simulink model "Custom_SP_inverse"  (R2020b)
settings: Solver=ode45  StartTime=0.0  StopTime=40  RelTol=1e-3
model workspace (MATLAB code in the model file):
  | %% PARAMETERS FOR CUSTOM_SP
  | %%%%%%%%%%%%%%%%%%%%% DENSITY %%%%%%%%%%%%%%%%%%%%%%%
  | al = 2.07; % g/cm^3
  | steel = 7.833; %g/cm^3
  | 
  | %%%%%%%%%%%%%%%%%%%%% BASE COORDINATES %%%%%%%%%%%%%%%%%%%%%%%
  | % Outside coordinates
  | out_base_right = [-335 -170.32; -315 -204.96;
  |     -315 -295.6; -98.49 -420.6; -20 -375.28;
  |     20 -375.28; 315 -204.96; 335 -170.32; 413.49 -125];
  | out_base_left = [413.49 125; 335 170.32;
  |     315 204.96; 20 375.28; -20 375.28;
  |     -98.49 420.6; -315 295.6; -315 204.96; -335 170.32;
  |     -335 -170.32];
  | out_base = [out_base_right; out_base_left];
  | 
  | % Inside coordinates
  | in_base = [-230 -246.52; -230 246.52; -98.49 322.45; 328.49 75.93;
  |     328.49 -75.93; -98.49 -322.45; -230 -246.52];
  | 
  | tot_base = [out_base; in_base];
  | 
  | %%%%%%%%%%%%%%%%%%%%%%% PLATE POSE ON BASE %%%%%%%%%%%%%%%%%%%%%%%%%%%
  | % PLATE POSITION ON BASE
  | plate_1 = [-272.22 -252.09 0];
  | plate_2 = [-82.21 -361.79 0];
  | plate_3 = [354.42 -109.71 0];
  | plate_4 = [354.42 109.71 0];
  | plate_5 = [-82.21 361.79 0];
  | plate_6 = [-272.22  252.09 0];
  | 
  | % ANGLE FOR JOINT ON BASE
  | plate_angle_1 = 0 + pi/2;
  | plate_angle_2 = 2*pi/3 + pi/2;
  | plate_angle_3 = 2*pi/3 + pi/2;
  | plate_angle_4 = 4*pi/3 + pi/2;
  | plate_angle_5 = 4*pi/3 + pi/2;
  | plate_angle_6 = 0 + pi/2;
  | 
  | %%%%%%%%%%%%%%%%%%%%%%%% FLANGE COORDINATES %%%%%%%%%%%%%%%%%%%%%%%%%%%%
  | flange_body = [ -20 22.5; -20 -22.5; 13.6488 -9.3106];
  | 
  | C = linspace(-68.6, 68.6, 21)';
  | C = deg2rad(C);
  | flange_round = [10+10*cos(C) 10*sin(C)];
  | 
  | C = linspace(3*pi/2, -pi/2, 100)';
  | flange_hole = [10+6*cos(C) 6*sin(C)];
  | 
  | flange = [flange_round; flange_body; flange_hole];
  | 
  | %plot(flange(:,1),flange(:,2), 'Color', [0.6 0.6 0.6], 'Marker', '.',...
  | %'MarkerSize', 9, 'MarkerEdgeColor', [1 0 0]);
  | 
  | %%%%%%%%%%%%%%%%%%%%%%%%%%%%% LID %%%%%%%%%%%%%%%%%%%%%%%%%%%%%%
  | % LID COORDINATES
  | C = linspace(-150 , -70, 9)';
  | C = deg2rad(C);
  | lid_round1 = [-171.37+10*cos(C) -103.18+10*sin(C)];
  | 
  | C = linspace(110, 60, 9)';
  | C = deg2rad(C);
  | lid_round2 = [-118.05+10*cos(C) -105.05+10*sin(C)];
  | 
  | C = linspace(60, 10, 9)';
  | C = deg2rad(C);
  | lid_round3 = [-117.46+10*cos(C) -105.39+10*sin(C)];
  | 
  | C = linspace(110, 60, 9)';
  | C = deg2rad(C);
  | lid_round4 = [-32.54+10*cos(C) -154.42+10*sin(C)];
  | 
  | C = linspace(60, 10, 9)';
  | C = deg2rad(C);
  | lid_round5 = [-31.95+10*cos(C) -154.76+10*sin(C)];
  | 
  | C = linspace(-90-80, -90, 9)';
  | C = deg2rad(C);
  | lid_round6 = [-3.67+10*cos(C) -200+10*sin(C)];
  | 
  | C = linspace(-30, 50, 9)';
  | C = deg2rad(C);
  | lid_round7 = [175.04+10*cos(C) -96.82+10*sin(C)];
  | 
  | C = linspace(-140, -90, 9)';
  | C = deg2rad(C);
  | lid_round8 = [150+10*sin(C) -49.71+10*cos(C)];
  | 
  | C = linspace(-90, -40, 9)';
  | C = deg2rad(C);
  | lid_round9 = [150+10*sin(C) -49.03+10*cos(C)];
  | 
  | C = linspace(-140, -90, 9)';
  | C = deg2rad(C);
  | lid_round10 = [150+10*sin(C) 49.03+10*cos(C)];
  | 
  | C = linspace(-90, -40, 9)';
  | C = deg2rad(C);
  | lid_round11 = [150+10*sin(C) 49.71+10*cos(C)];
  | 
  | C = linspace(-50, 30, 9)';
  | C = deg2rad(C);
  | lid_round12 = [175.04+10*cos(C) 96.82+10*sin(C)];
  | 
  | C = linspace(90, 90+80, 9)';
  | C = deg2rad(C);
  | lid_round13 = [-3.67+10*cos(C) 200+10*sin(C)];
  | 
  | C = linspace(-10, -60, 9)';
  | C = deg2rad(C);
  | lid_round14 = [-31.95+10*cos(C) 154.76+10*sin(C)];
  | 
  | C = linspace(-60, -110, 9)';
  | C = deg2rad(C);
  | lid_round15 = [-32.54+10*cos(C) 154.42+10*sin(C)];
  | 
  | C = linspace(-10, -60, 9)';
  | C = deg2rad(C);
  | lid_round16 = [-117.46+10*cos(C) 105.39+10*sin(C)];
  | 
  | C = linspace(-60, -110, 9)';
  | C = deg2rad(C);
  | lid_round17 = [-118.05+10*cos(C) 105.05+10*sin(C)];
  | 
  | C = linspace(70 , 150, 9)';
  | C = deg2rad(C);
  | lid_round18 = [-171.37+10*cos(C) 103.18+10*sin(C)];
  | 
  | lid = [-200 -73.59; lid_round1; lid_round2;
  |     lid_round3;
  |     -100.49 -144.05; -74.51 -159.05; lid_round4;
  |     lid_round5; lid_round6; 36.27 -210; 163.73 -136.41;
  |     lid_round7; lid_round8; lid_round9; 175 -15; 175 15;
  |     lid_round10; lid_round11; lid_round12; 163.73 136.41;
  |     36.27 210; lid_round13; lid_round14; lid_round15;
  |     -74.51 159.05; -100.49 144.05; lid_round16;
  |     lid_round17; lid_round18; -200 73.59];
  | 
  | lid = [-200 -73.59; lid_round1; lid_round2; lid_round3;
  |     -100.49 -144.05; -74.51 -159.05;
  |     lid_round4; lid_round5; lid_round6;
  |     36.27 -210; 163.73 -136.41;
  |     lid_round7; lid_round8; lid_round9;
  |     175 -15; 175 15;
  |     lid_round10; lid_round11; lid_round12;
  |     163.73 136.41; 36.27 210;
  |     lid_round13; lid_round14; lid_round15;
  |     -74.51 159.05; -100.49 144.05;
  |     lid_round16; lid_round17; lid_round18; -200 73.59];
  | 
  | % LID CONNECTOR
  | C = linspace(-150 , -50, 15)';
  | C = deg2rad(C);
  | lid_connector_round1 = [2.15+10*cos(C) -79.37+10*sin(C)];
  | 
  | C = linspace(-50 , 0, 15)';
  | C = deg2rad(C);
  | lid_connector_round2 = [37.5+10*cos(C) -49.71+10*sin(C)];
  | 
  | C = linspace(0 , 50, 15)';
  | C = deg2rad(C);
  | lid_connector_round3 = [37.5+10*cos(C) -49.03+10*sin(C)];
  | 
  | C = linspace(-50, 0, 15)';
  | C = deg2rad(C);
  | lid_connector_round4 = [37.5+10*cos(C) 49.03+10*sin(C)];
  | 
  | C = linspace(0, 50, 15)';
  | C = deg2rad(C);
  | lid_connector_round5 = [37.5+10*cos(C) 49.71+10*sin(C)];
  | 
  | C = linspace(50 , 150, 15)';
  | C = deg2rad(C);
  | lid_connector_round6 = [2.15+10*cos(C) 79.37+10*sin(C)];
  | 
  | lid_connector = [-12.5 -74; lid_connector_round1;
  |     lid_connector_round2; lid_connector_round3; 12.5 -15;
  |     12.5 15; lid_connector_round4; lid_connector_round5;
  |     lid_connector_round6; -12.5 74];
  | 
  | %%%%%%%%%%%%%%%%%%%%%%%%% BALL JOINT %%%%%%%%%%%%%%%%%%%%%%%%%%%
  | % BALL JOINTS
  | C = linspace(138.59, 41.41, 50)';
  | C = deg2rad(C);
  | ball_round = [10*sin(C) 10*cos(C)];
  | 
  | ball_joint = [6 -7.5; ball_round; 6 7.5];
  | 
  | % BALL CONNECTOR
  | C = linspace(-109.47, -70.53, 49)';
  | C = deg2rad(C);
  | ball_round_out = [-16*sin(C) 16*cos(C)];
  | 
  | C = linspace(-57.75, -122.25, 49)';
  | C = deg2rad(C);
  | ball_round_in = [-10*sin(C) 10*cos(C)];
  | 
  | ball_connector = [ball_round_out; ball_round_in];
  | 
  | %%%%%%%%%%%%%%%%%%%%%%%%%% MOTOR %%%%%%%%%%%%%%%%%%%%%%%%%%%
  | % KNOB UNDER MOTOR
  | C = linspace(-90+25.84, -90+64.16, 50)';
  | C = deg2rad(C);
  | knob_under_round1 = [7.5*sin(C) -7.5*cos(C)];
  | 
  | C = linspace( -64.16, -25.84, 50)';
  | C = deg2rad(C);
  | knob_under_round2 = [7.5*cos(C) 7.5*sin(C)];
  | 
  | C = linspace( 25.84, 64.16, 50)';
  | C = deg2rad(C);
  | knob_under_round3 = [7.5*cos(C) 7.5*sin(C)];
  | 
  | C = linspace( 64.16, 25.84, 50)';
  | C = deg2rad(C);
  | knob_under_round4 = [-7.5*cos(C) 7.5*sin(C)];
  | 
  | knob_under = [knob_under_round1; knob_under_round2;
  |     knob_under_round3; knob_under_round4];
  | 
  | % MOTOR UNDER
  | C = linspace(-90, -49, 10)';
  | C = deg2rad(C);
  | knob_under_round1 = [-(19+17)+5.5*sin(C) -11.13-5.5*cos(C)];
  | 
  | C = linspace(-49, 0, 10)';
  | C = deg2rad(C);
  | knob_under_round2 = [-(17+14.77)+5.5*sin(C) -16-5.5*cos(C)];
  | 
  | C = linspace(0, 180, 49)';
  | C = deg2rad(C);
  | knob_under_round3 = [20+21.5*sin(C) -21.5*cos(C)];
  | 
  | C = linspace(180, 180+49, 10)';
  | C = deg2rad(C);
  | knob_under_round4 = [-(17+14.77)+5.5*sin(C) 16-5.5*cos(C)];
  | 
  | C = linspace(270-49, 270, 10)';
  | C = deg2rad(C);
  | knob_under_round5 = [-(19+17)+5.5*sin(C) 11.13-5.5*cos(C)];
  | 
  | motor_under = [knob_under_round1; knob_under_round2;
  |     knob_under_round3; knob_under_round4; knob_under_round5];
  | 
  | % MOTOR LINEAR
  | C = linspace(-180, -101.99, 10)';
  | C = deg2rad(C);
  | motor_top_round1 = [-15.28+3*cos(C) -8.62+3*sin(C)];
  | 
  | C = linspace(-101.99, 101.99, 49)';
  | C = deg2rad(C);
  | motor_top_round2 = [3.12+15.25*cos(C) 15.25*sin(C)];
  | 
  | C = linspace(101.99, 180, 10)';
  | C = deg2rad(C);
  | motor_top_round3 = [-15.28+3*cos(C) 8.62+3*sin(C)];
  | 
  | C = linspace(180, -180, 50)';
  | C = deg2rad(C);
  | motor_top_hole = [3.12+10.1*cos(C) 10.1*sin(C)];
  | 
  | motor_linear = [motor_top_round1; motor_top_round2; motor_top_round3;
  |     -15.28-3 -8.62; motor_top_hole];
  | 
  | %%%%%%%%%%%%%%%%%%%%% MALE %%%%%%%%%%%%%%%%%%%%%%%%%%%
  | male = [15.1 -16; 15.1 16; 10.1 16;
  |     10.1 -11; 6 -11; 6 -16];
  | 
  | %%%%%%%%%%%%%%%%%%%%% FEMALE %%%%%%%%%%%%%%%%%%%%%%%%%
  | female = [15 -19; 15 19; 9.5 19; 9.5 1;
  |     5.055 1; 5.055 -19];
  | 
  | %%%%%%%%%%%%%%%%%%%%% STRAIN GAUGE %%%%%%%%%%%%%%%%%%%%%%
  | strain_gauge = [-38.1 -25.4; -22.4 -25.4; -22.4 11.6;
  |     -13.9 11.6; -13.9 -25.4; 38.1 -25.4; 38.1 25.4;
  |     22.4 25.4; 22.4 -11.6; 13.9 -11.6;
  |     13.9 25.4; -38.1 25.4];
  | 
  | %%%%%%%%%%%%%%%%%%%%% M12 STUFF %%%%%%%%%%%%%%%%%%%%%%%%%%%
  | % M12 BOLT
  | m12_bolt = [0 -18.5; 6 -18.5; 6 11.5; 10.1 11.5; 10.1 18.5; 0 18.5];
  | 
  | % M12 NUT
  | C = linspace(3*pi, pi, 50)';
  | m12_hole = [6*cos(C) 6*sin(C)];
  | m12_nut = [-21.2/2 0; -5.48 -9.5; 5.48 -9.5; 21.2/2 0; 5.48 9.5; -5.48 9.5; -21.2/2 0; m12_hole];
  | 
  | % M12 WASHER
  | m12_washer = [6 -1; 23.5/2 -1; 23.5/2 1; 6 1];
  | 
  | %%%%%%%%%%%%%%%%%%%%%% PLATFORM COORDINATES %%%%%%%%%%%%%%%%%%%%%%%%%%%
  | % Outside coordinates
  | out_platform = [36.27 -210; 163.73 -136.41;
  |     200 -73.59; 200 73.59; 163.73 136.41;
  |     36.27 210; -36.27 210; -163.73 136.41;
  |     -200 73.59; -200 -73.54; -163.73 -136.41; -36.27 -210;
  |     36.27 -210];
  | C = linspace(3*pi/2, -pi/2, 100)';
  | platform_hole = [140*cos(C) 140*sin(C)];
  | platform = [out_platform; platform_hole];
  | 
  | %%%%%%%%%%%%%%%%%%%% STUMP %%%%%%%%%%%%%%%%%%%%%%%
  | C = linspace(-pi/2, -deg2rad(12.47), 100)';
  | stump_round = [70*cos(C) -100+70*sin(C)];
  | stump = [stump_round; 100 170; 0 170];
  | 
  | %% POSITION OF BASE JOINT AND PLATFORM JOINT FOR INVERSE KINEMATICS
  | % BASE JOINT POSITION
  | 
  | zb = 5 + 5 + 30;
  | B = [plate_1(1,1:2) zb; plate_2(1,1:2) zb; plate_3(1,1:2) zb; plate_4(1,1:2) zb; plate_5(1,1:2) zb; plate_6(1,1:2) zb]';
  | 
  | 
  | % JOINT POSITION ON PLATFORM
  | Rot = [cos(deg2rad(120)) -sin(deg2rad(120)); sin(deg2rad(120)) cos(deg2rad(120))];
  | platform_joint_1 = [-200.54-18.5 -48.83]';
  | platform_joint_6 = [-200.54-18.5 48.83]';
  | platform_joint_2 = Rot*platform_joint_6;
  | platform_joint_3 = Rot*platform_joint_1;
  | platform_joint_4 = Rot*platform_joint_2;
  | platform_joint_5 = Rot*platform_joint_3;
  | 
  | % LEG LENGHT AT HOME POSITION
  | %ball_joint_bottom_length = 13.75; %mm
  | %nut_washer = 10 + 2 + 7.25; %mm
  | %female_length = 38 + 2; %mm
  | %motor_length = 58.5 + 163.5; %mm
  | %extender_length = 20 + 50; %mm
  | %male_bolt_nut = 5 + 7 + 25; %mm
  | %strain_gauge_length = 38.1*2; %mm
  | %nut = 10 + 7.25; %mm
  | %ball_joint_top_length = 13.75; %mm
  | 
  | %leg_initial_length = ball_joint_bottom_length + nut_washer + female_length + motor_length + extender_length + male_bolt_nut + strain_gauge_length + nut + ball_joint_top_length;
  | 
  | %height_home = sqrt(leg_initial_length^2 - (plate_1(1)-platform_joint_1(1))^2 - (plate_1(2)-platform_joint_1(2))^2)+zb;
  | height_home = 503.318 + 2.5;
  | leg_initial_length = sqrt((plate_1(1)-platform_joint_1(1))^2 + (plate_1(2)-platform_joint_1(2))^2 + (height_home-zb)^2);
  | P = [platform_joint_1' height_home; platform_joint_2' height_home; platform_joint_3' height_home; platform_joint_4' height_home; platform_joint_5' height_home; platform_joint_6' height_home]';
libraries: nesl_utility x19, Custom_SP_lib x8, sm_lib x2
(part 1 of 2)
settings Model: Creator=ellen  LastModifiedBy=ellen
settings DataIOCC: LimitDataPoints=on

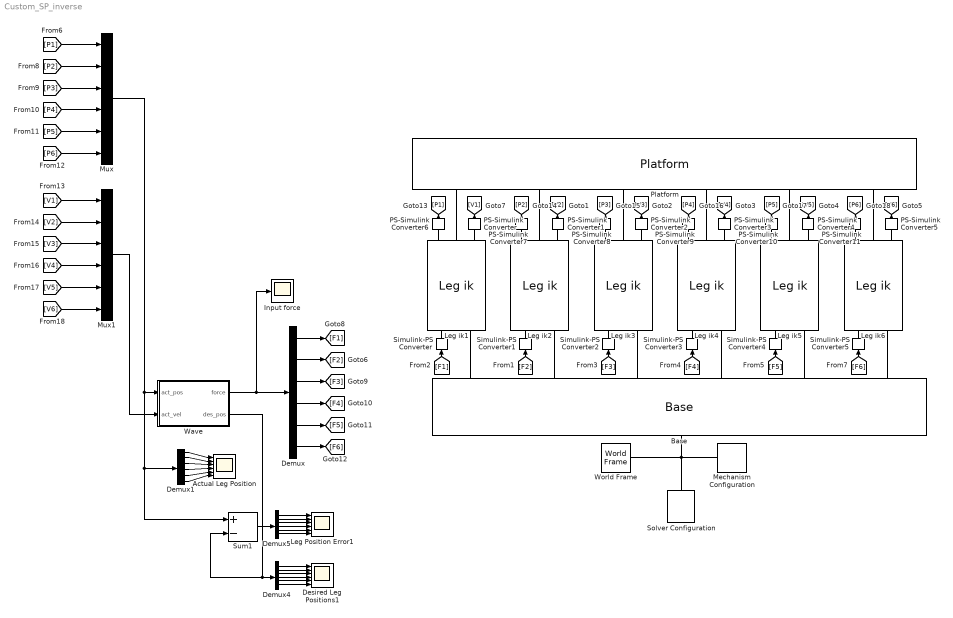
== system Custom_SP_inverse ==
  Actual Leg Position : Scope  NumInputPorts=6
  Base : Custom_SP_lib/Base  SystemSampleTime=-1  VariantActivationTime=update diagram  Latency=0  AutoFrameSizeCalculation=off
  Demux{,1,4..5} (4 alike) : Demux  Outputs=6
  Desired Leg Positions1 : Scope  NumInputPorts=6
  Input force : Scope
  Leg Position Error1 : Scope  NumInputPorts=6
  Leg ik1 : Custom_SP_lib/Leg ik  SystemSampleTime=-1  VariantActivationTime=update diagram  Latency=0  AutoFrameSizeCalculation=off
      link override Motor ik1: leg_offset=0
      link override Motor ik1/Actuation: PositionTargetValue=0
  Leg ik2 : Custom_SP_lib/Leg ik  SystemSampleTime=-1  VariantActivationTime=update diagram  Latency=0  AutoFrameSizeCalculation=off
      link override Motor ik1: leg_offset=0
      link override Motor ik1/Actuation: PositionTargetValue=0
  Leg ik3 : Custom_SP_lib/Leg ik  SystemSampleTime=-1  VariantActivationTime=update diagram  Latency=0  AutoFrameSizeCalculation=off
      link override Motor ik1: leg_offset=0
      link override Motor ik1/Actuation: PositionTargetValue=0
  Leg ik4 : Custom_SP_lib/Leg ik  SystemSampleTime=-1  VariantActivationTime=update diagram  Latency=0  AutoFrameSizeCalculation=off
      link override Motor ik1: leg_offset=0
      link override Motor ik1/Actuation: PositionTargetValue=0
  Leg ik5 : Custom_SP_lib/Leg ik  SystemSampleTime=-1  VariantActivationTime=update diagram  Latency=0  AutoFrameSizeCalculation=off
      link override Motor ik1: leg_offset=0
      link override Motor ik1/Actuation: PositionTargetValue=0
  Leg ik6 : Custom_SP_lib/Leg ik  SystemSampleTime=-1  VariantActivationTime=update diagram  Latency=0  AutoFrameSizeCalculation=off
      link override Motor ik1: leg_offset=0
      link override Motor ik1/Actuation: PositionTargetValue=0
  Mechanism Configuration : sm_lib/Utilities/Mechanism Configuration  UniformGravity=Constant  GravityVector=[0 0 -9.81]  GravityVectorUnits=m/s^2  GravityUnits=m/s^2  LinearizationDelta=0.001  JointModeTransitionNonlinearIterations=2
  Mux : Mux  Inputs=6
  Mux1 : Mux  Inputs=6
  PS-Simulink Converter{,1..5} (6 alike) : nesl_utility/PS-Simulink Converter  PhysicalDomain=network_engine_domain  SubClassName=ps_output  LeftPortType=input  RightPortType=output  PseudoPeriodic=off  Frequencies=[]  Unit=mm/s  AffineConversion=off
  PS-Simulink Converter{6..11} (6 alike) : nesl_utility/PS-Simulink Converter  PhysicalDomain=network_engine_domain  SubClassName=ps_output  LeftPortType=input  RightPortType=output  PseudoPeriodic=off  Frequencies=[]  Unit=mm  AffineConversion=off
  Platform : Custom_SP_lib/Platform  SystemSampleTime=-1  VariantActivationTime=update diagram  Latency=0  AutoFrameSizeCalculation=off
  Simulink-PS Converter{,1..5} (6 alike) : nesl_utility/Simulink-PS Converter  PhysicalDomain=network_engine_domain  SubClassName=ps_input  LeftPortType=input  RightPortType=output  PseudoPeriodic=off  Frequencies=[]  NoiseDistribution=none  NoiseParameters=[]  Unit=1  AffineConversion=off  FilteringAndDerivatives=provide  SimscapeFilterOrder=1  InputFilterTimeConstant=0.001  UdotUserProvided=0
  Solver Configuration : nesl_utility/Solver Configuration  PhysicalDomain=network_engine_domain  SubClassName=solver  LeftPortType=input  RightPortType=generic  Tones=[]  Harmonics=[]  SimulateNoise=off  Profile=off  UseLocalSampling=off  EnableSwitchedLinearOptims=on  FrequencyDomain=off  UseCCode=off  RelTol=0.001  AbsTol=1e-06  MinStep=1e-09  ToWorkspace=off  RevertToSquareIcSolve=off  NumHomotopyIterations=100  PhasorMode=off  PhasorModeNumHarmonics=1  DoDC=off  ResidualTolerance=1e-9  UseLocalSolver=off  LocalSolverChoice=NE_BACKWARD_EULER_ADVANCER  LocalSolverSampleTime=.001  DoFixedCost=off  MaxNonlinIter=3  MaxModeIter=2  ComputeImpulses=off  ImpulseIterations=2  LinearAlgebra=Sparse  EquationFormulation=NE_TIME_EF  DelaysMemoryBudget=1024  AutomaticFiltering=on  FilteringTimeConstant=0.001  PartitionStorageMethod=AS_NEEDED  PartitionMemoryBudget=1024  PartitionMethod=FAST
  Sum1 : Sum  Inputs=+-
  Wave : Subsystem
  World Frame : sm_lib/Frames and Transforms/World Frame
  wires:
  PS-Simulink Converter5/1 -> [V6]
  PS-Simulink Converter1/1 -> [V2]
  PS-Simulink Converter3/1 -> [V4]
  PS-Simulink Converter/1 -> [V1]
  [P2] -> Mux/2
  [P1] -> Mux/1
  [P6] -> Mux/6
  [P4] -> Mux/4
  [P5] -> Mux/5
  PS-Simulink Converter4/1 -> [V5]
  [P3] -> Mux/3
  PS-Simulink Converter2/1 -> [V3]
  Demux/5 -> [F5]
  Demux/4 -> [F4]
  Demux/1 -> [F1]
  Demux/3 -> [F3]
  Demux/2 -> [F2]
  Demux/6 -> [F6]
  [V4] -> Mux1/4
  [V6] -> Mux1/6
  [V2] -> Mux1/2
  [V5] -> Mux1/5
  [V1] -> Mux1/1
  [V3] -> Mux1/3
  PS-Simulink Converter6/1 -> [P1]
  PS-Simulink Converter7/1 -> [P2]
  PS-Simulink Converter8/1 -> [P3]
  PS-Simulink Converter9/1 -> [P4]
  PS-Simulink Converter10/1 -> [P5]
  PS-Simulink Converter11/1 -> [P6]
  [F1] -> Simulink-PS Converter/1
  [F2] -> Simulink-PS Converter1/1
  [F3] -> Simulink-PS Converter2/1
  [F4] -> Simulink-PS Converter3/1
  [F5] -> Simulink-PS Converter4/1
  [F6] -> Simulink-PS Converter5/1
  Demux1/1 -> Actual Leg Position/1
  Demux1/2 -> Actual Leg Position/2
  Demux1/3 -> Actual Leg Position/3
  Demux1/4 -> Actual Leg Position/4
  Demux1/5 -> Actual Leg Position/5
  Demux1/6 -> Actual Leg Position/6
  Mux/1 -> Demux1/1, Sum1/1, Wave/1(act_pos)
  Mux1/1 -> Wave/2(act_vel)
  Wave/1(force) -> Demux/1, Input force/1
  Wave/2(des_pos) -> Sum1/2, Demux4/1
  Demux4/3 -> Desired Leg Positions1/3
  Demux4/4 -> Desired Leg Positions1/4
  Demux4/6 -> Desired Leg Positions1/6
  Demux4/1 -> Desired Leg Positions1/1
  Demux4/5 -> Desired Leg Positions1/5
  Demux4/2 -> Desired Leg Positions1/2
  Demux5/4 -> Leg Position Error1/4
  Demux5/2 -> Leg Position Error1/2
  Demux5/3 -> Leg Position Error1/3
  Demux5/1 -> Leg Position Error1/1
  Demux5/6 -> Leg Position Error1/6
  Demux5/5 -> Leg Position Error1/5
  Sum1/1 -> Demux5/1
  connections:
  Solver Configuration/RConn1 -- World Frame/RConn1 -- Base/RConn1 -- Mechanism Configuration/RConn1
  Leg ik3/RConn3 -- PS-Simulink Converter2/LConn1
  Leg ik1/RConn3 -- PS-Simulink Converter/LConn1
  Leg ik6/RConn3 -- PS-Simulink Converter5/LConn1
  Leg ik5/RConn3 -- PS-Simulink Converter4/LConn1
  Leg ik2/RConn3 -- PS-Simulink Converter1/LConn1
  Leg ik4/RConn3 -- PS-Simulink Converter3/LConn1
  Leg ik2/RConn2 -- Platform/RConn2
  Leg ik6/RConn2 -- Platform/RConn6
  Leg ik1/LConn2 -- Base/LConn1
  Leg ik5/RConn2 -- Platform/RConn5
  Base/LConn2 -- Leg ik2/LConn2
  Leg ik4/RConn2 -- Platform/RConn4
  Leg ik5/LConn2 -- Base/LConn5
  Leg ik3/LConn2 -- Base/LConn3
  Leg ik4/LConn2 -- Base/LConn4
  Base/LConn6 -- Leg ik6/LConn2
  Leg ik3/RConn2 -- Platform/RConn3
  Leg ik1/RConn2 -- Platform/RConn1
  Leg ik1/RConn1 -- PS-Simulink Converter6/LConn1
  Leg ik2/RConn1 -- PS-Simulink Converter7/LConn1
  Leg ik3/RConn1 -- PS-Simulink Converter8/LConn1
  Leg ik4/RConn1 -- PS-Simulink Converter9/LConn1
  Leg ik5/RConn1 -- PS-Simulink Converter10/LConn1
  Leg ik6/RConn1 -- PS-Simulink Converter11/LConn1
  Leg ik1/LConn1 -- Simulink-PS Converter/RConn1
  Leg ik2/LConn1 -- Simulink-PS Converter1/RConn1
  Leg ik3/LConn1 -- Simulink-PS Converter2/RConn1
  Leg ik4/LConn1 -- Simulink-PS Converter3/RConn1
  Leg ik5/LConn1 -- Simulink-PS Converter4/RConn1
  Leg ik6/LConn1 -- Simulink-PS Converter5/RConn1

== system Custom_SP_inverse/Wave ==
  act_pos : Inport
  act_vel : Inport  Port=2
  Controller : Subsystem  mask(PID Controller){Kp=300, Ki=20, Kd=5}
      mask prompts: Kp "Proportional Gain"; Ki "Integral Gain"; Kd "Derivative Gain"
      mask help:
      | Generates an actuation output based on a desired trajectory and an actual trajectory, using a generic proportional-integral-derivative (PID) control law.  The three control gains are specified through parameters.
      |
      | Both the desired and actual trajectories are specified by separate position and velocity input signals.  The controller is generic and can control to trajectories through state spaces of arbitrary dimension; the only requirement is that all four inputs have the same dimension.
      mask Help:
      | A <em>PID Controller</em> generates an actuation output based on a desired trajectory and an actual trajectory, using a generic proportional-integral-derivative (PID) control law.  The three control gains are specified through parameters.
      | 
      | Both the desired and actual trajectories are specified by separate position and velocity input signals.  The controller is generic and can control to trajectories through state spaces of arbitrary dimension; the only requirement is that all four inputs have the same dimension.
      | 
      | This block is not specific to the Stewart platform and could serve in any general purpose control library.  For the Stewart platform application, the trajectories are all through the 6-D leg-position space.
      | 
      | <h3>Gains</h3>
      | 
      | The parameters specify the gains of the controller.
      | 
      | <ul>
      | 
      | <li> <b>Proportional Gain</b> The gain that determines the strength of the control actuation in response to current deviations between actual and desired positions.  This affects the responsiveness of the controller but can lead to instability if set too high.
      | 
      | <li> <b>Integral Gain</b> The gain that determines the strength of the control actuation in response to deviations between actual and desired positions that persist over time.  A nonzero integral term is often necessary to avoid <em>droop</em> (steady-state error).  Higher values reduce the transient response of the controller but can cause overshoot in the controlled position.
      | 
      | <li> <b>Derivative Gain</b> The gain that determines the strength of the control actuation in response to the derivative of the deviations between actual and desired positions.  This is a damping component used to reduce overshoot in the controlled position; the tradeoff is that it reduces the transient response of the controller.  Higher values increase the stiffness of the system and can lead to instability.
      | 
      | </ul>
      | 
      | 
      | <h3>Ports</h3>
      | 
      | <ul>
      | 
      | <li> <b>act_pos</b> The current actual position of the plant.
      | 
      | <li> <b>act_pos</b> The current actual velocity of the plant.  This should be the time derivative of the <em>act_pos</em> signal.
      | 
      | <li> <b>des_pos</b> The current desired position of the plant.
      | 
      | <li> <b>des_pos</b> The current desired velocity of the plant.  This should be the time derivative of the <em>des_pos</em> signal.
      | 
      | </ul>
  Inverse Kinematics Module : Subsystem  mask(Stewart Platform Inverse Kinematics){}
      mask help:
      | Performs the essential inverse kinematic computations for a Stewart platform manipulator.
      |
      | Given a desired dynamic state of a Stewart platform manipulator specified by a 3-D rigid transformation from the gripper frame to the base reference frame, and the first time derivative of this transformation, this block computes the positions and velocities of the prismatic primitives of the six cylindrical leg joints necessary to achieve the desired dynamic state.
      mask Help:
      | A <em>Stewart Platform Inverse Kinematics</em> performs the essential inverse kinematic computations for a Stewart platform manipulator.
      | 
      | Given a desired dynamic state of a Stewart platform manipulator specified by a 3-D rigid transformation from the gripper frame to the base reference frame, and the first time derivative of this transformation, this block computes the positions and velocities of the prismatic primitives of the six cylindrical leg joints necessary to achieve the desired dynamic state.
      | 
      | <h3>Manipulator Transformation</h3>
      | 
      | The desired dynamic state of a Stewart platform manipulator may be specified by a single 3-D rigid transformation, called the <em>manipulator transformation</em>, and its time derivative.  The transformation is from <em>gripper</em> frame to <em>base</em> frame coordinates.  The base frame is attached to the base plate of the manipulator.  Its origin is located at the center of the base, and the z-axis points directly upward.  The gripper frame is located somewhere directly above the center of platform plate of the manipulator, and is aligned with the base frame when the positions of the prismatic primitives of all six cylindrical leg joints are equal.
      | 
      | In the following discussions, let <b>R</b> and <b>d</b> specify the rotation matrix and displacement vector, respectively, of the manipulator transformation. That is, <b>d</b> is the origin of the gripper frame specified in base frame coordinates, and the columns of <b>R</b> are the canonical <b>i</b>, <b>j</b>, and <b>k</b> vectors of the gripper frame resolved in base frame coordinates.
      | Let <b>R'</b> and <b>d'</b> be the first time derivatives of <b>R</b> and <b>d</b>, respectively.
      | 
      | <h3>Inverse Kinematics</h3>
      | 
      | Each of the six legs of the manipulator is attached between a pair of universal joints: one on the base plate and one on the platform plate.  Each leg has an internal knee joint with a sensed and actuated prismatic primitive.
      | Let <em>q_i</em> and <em>q_i'</em> be the position and velocity of this primitive on Leg <em>i</em>.  Let <em>L0</em> denote the <em>nominal</em> lengths of the legs.  This is the length of a leg when its prismatic primitive is at the zero position.
      | 
      | The goal of the inverse kinematics computation is to determine the values of <em>q_i</em> and <em>q_i'</em> for i = 1, ..., 6 needed to achieve a particular manipulator transformation and its derivative.
      | 
      | The key to understanding the inverse kinematics computations is to consider the positions of the centers of the pairs of universal joints.  (These points are the centers of the crosspieces visible in the visualization of the manipulator.)
      | 
      | Let <b>b</b>_i and <b>p</b>_i be the 3-D points specifying the center of the universal joints on the base and platform plates, respectively, to which Leg <em>i</em> is connected. <b>b</b>_i is specified in base frame coordinates, and <b>p</b>_i is specified in gripper frame coordinates.  Then the desired position of the prismatic primitive of the knee joint of Leg <em>i</em> is given by
      | 
      | <em>q_i</em> = || <b>R</b> <b>p</b>_i + <b>d</b> - <b>b</b>_i || - <em>L0</em>.
      | 
      | Denote the vector within the norm expression above as <b>o</b>_i (<b>o</b> for <em>offset</em>).
      | 
      | The desired velocity of the prismatic primitive of the knee joint of Leg <em>i</em> is obtained by differentiating the expression for <em>q_i</em>. Noting that <b>p</b>_i, <b>b</b>_i, and <em>L0</em> are constant, the result is:
      | 
      | <em>q_i'</em> = [ (<b>R'</b> <b>p</b>_i + <b>d'</b>) . <b>o</b>_i ] / || <b>o</b>_i ||.
      | 
      | Note that the denominator of this expression is equal to the vector norm in the expression for <em>q_i</em>.
      | 
      | This block computes the values of all six prismatic primitive positions and velocities according to the expressions above.  The computation of the (constant) <b>p</b>_i and <b>b</b>_i points is highly dependent on the manipulator kinematics and done in the mask initialization of the containing <em>Stewart Platform System</em> block.
      | 
      | <h3>Ports</h3>
      | 
      | <ul>
      | 
      | <li> <b>d</b> The displacement vector of the desired manipulator transformation (see above) in units of centimeters.
      | 
      | <li> <b>R</b> The rotation matrix of the desired manipulator transformation (see above).
      | 
      | <li> <b>d'</b> The time derivative of the displacement vector of the desired manipulator transformation in units of centimeters/second.
      | 
      | <li> <b>R'</b> The time derivative of the rotation matrix of the desired manipulator transformation.
      | 
      | <li> <b>pos</b> The computed positions of the prismatic primitives of the six leg joints, as a 6 x 1 vector in units of centimeters.
      | 
      | <li> <b>vel</b> The computed velocities of the prismatic primitives of the six leg joints, as a 6 x 1 vector in units of centimeters/second.
      | 
      | 
      | </ul>
      | 
      | <!--  LocalWords:  ith pos vel
      |  -->
  Reference Trajectory Generator1 : Subsystem  mask(3-D Transform Trajectory Generator){Ax=0, wx=0, px=0, kx=0, Ay=0, wy=0, py=0, ky=0, Az=30, wz=180/10, pz=-90, kz=0, Aa=3, wa=360*3/10, pa=0, ka=0, Ab=3, wb=360*3/10, pb=-90, kb=0, Ac=0, wc=0, pc=0, kc=0}
      mask prompts: Ax "X Displacement Amplitude (mm)"; wx "X Displacement Frequency (deg / s)"; px "X Displacement Phase (deg)"; kx "X Displacement Offset (mm)"; Ay "Y Displacement Amplitude (mm)"; wy "Y Displacement Frequency (deg / s)"; py "Y Displacement Phase (deg)"; ky "Y Displacement Offset (mm)"; Az "Z Displacement Amplitude (mm)"; wz "Z Displacement Frequency (deg / s)"; pz "Z Displacement Phase (deg)"; kz "Z Displacement Offset (mm)"; Aa "X Rotation Amplitude (deg)"; wa "X Rotation Frequency (deg / s)"; pa "X Rotation Phase (deg)"; ka "X Rotation Offset (deg)"; Ab "Y Rotation Amplitude (deg)"; wb "Y Rotation Frequency (deg / s)"; pb "Y Rotation Phase (deg)"; kb "Y Rotation Offset (deg)"; Ac "Z Rotation Amplitude (deg)"; wc "Z Rotation Frequency (deg / s)"; pc "Z Rotation Phase (deg)"; kc "Z Rotation Offset (deg)"
      mask help: Tool for generating a wide variety of trajectories for a time-varying, 3-D rigid transformation between two frames.
      mask Help:
      | A <em>3-D Transform Trajectory Generator</em> is a tool for generating a wide variety of trajectories for a time-varying, 3-D rigid transformation between two frames.
      | 
      | A rigid transformation between two frames is characterized by a displacement vector and a rotation matrix.  Each of these can be parameterized with three scalar coordinates.  This block allows these six scalar coordinates to be parametrically specified as arbitrary sinusoidal functions of time.  The resulting displacement vector and rotation matrix, and their first derivatives are provided on the output ports.
      | 
      | <h3>Sinsoidal Functions</h3>
      | 
      | An arbitrary sinusoidal function of time is given by
      | 
      |     f(t) = A sin (w t + p) + k,
      | 
      | where <em>t</em> is time, and <em>A, w, p,</em> and <em>k</em> are scalar constants with the following meanings:
      | <ul>
      | <li> <em>A</em> is the <em>amplitude</em> of the sinusoid.
      | <li> <em>w</em> is the <em>angular frequency</em> of the sinusoid.
      | <li> <em>p</em> is the <em>phase</em> of the sinusoid.
      | <li> <em>k</em> is the <em>offset</em> of the sinusoid.
      | </ul>
      | 
      | <h3>Rigid Transformations</h3>
      | 
      | The time-varying, 3-D rigid transformation provided on the output ports of this block is, in turn, a function of scalar functions.  The displacement vector of the rigid transformation is given by:
      | 
      |     <b>d</b>(t) = [ x(t), y(t), z(t) ]^T
      | 
      | where x(t), y(t), and z(t) are scalar functions of time.
      | 
      | The rotation matrix of the rigid transformation is given by:
      | 
      |     <b>R</b>(t) = <b>R_x</b>(a(t)) <b>R_y</b>(b(t)) <b>R_z</b>(c(t)),
      | 
      | where a(t), b(t), and c(t) are scalar functions of time, and <b>R_x</b>, <b>R_y</b>, and <b>R_z</b> are rotations about the x, y, and z axes, respectively.
      | 
      | Note that this is an Euler angle parameterization of rotation.  The final rotation maps directions from a rotating frame F to a fixed frame G.  Beginning with F and G in an aligned configuration, the full rotation can be realized as a sequence of three rotations: first rotate F about its x-axis, then rotate F about its y-axis, and finally rotate F about its z-axis.  Alternatively, the rotation can be realized in a fixed-frame manner: first rotate F about G's z-axis, then rotate F about G's y-axis, and finally rotate F about G's z-axis. Both interpretations are correct.
      | 
      | The six scalar functions x(t), y(t), z(t), a(t), b(t), and c(t) are all arbitrary sinusoidal functions.  Each is parameterized by the four constants described in the preceding section.  This block computes these functions, and uses them to build the displacement vector, the rotation matrix, and the first time derivatives of these quantities.
      | 
      | 
      | <h3>Parameters</h3>
      | 
      | Each of the six parameter tabs defines four scalar parameters that together specify an arbitrary sinusoidal function of time, as described above.  The six tabs are:
      | 
      | <ul>
      | 
      | <li> <b>dx</b> Specifies the x-component of the displacement vector as a sinusoidal function of time.
      | 
      | <li> <b>dy</b> Specifies the y-component of the displacement vector as a sinusoidal function of time.
      | 
      | <li> <b>dz</b> Specifies the z-component of the displacement vector as a sinusoidal function of time.
      | 
      | <li> <b>Rx</b> Specifies the scalar rotation about the x-axis, part of the three-stage rotation sequence, as a sinusoidal function of time.
      | 
      | <li> <b>Ry</b> Specifies the scalar rotation about the y-axis, part of the three-stage rotation sequence, as a sinusoidal function of time.
      | 
      | <li> <b>Rz</b> Specifies the scalar rotation about the z-axis, part of the three-stage rotation sequence, as a sinusoidal function of time.
      | 
      | </ul>
      | 
      | <h3>Ports</h3>
      | 
      | <ul>
      | 
      | 
      | <li><b>d</b> The displacement vector of the time-varying, 3-D rigid transformation as a signal output.  This value is a 3 x 1 vector in units of centimeters.
      | 
      | <li><b>R</b> The rotation matrix of the time-varying, 3-D rigid transformation as a signal output.  This value is a 3 x 3 orthogonal matrix with +1 determinant.
      | 
      | <li><b>d'</b> The first time derivative of the signal appearing on the <em>d</em> port: a 3 x 1 vector in units of centimeters/second.
      | 
      | <li><b>R'</b> The first time derivative of the signal appearing on the <em>R</em> port: a 3 x 3 matrix.
      | 
      | </ul>
      mask DialogControl ParameterTabVar0 Prompt: dx
      mask DialogControl ParameterTabVar01 Prompt: dy
      mask DialogControl ParameterTabVar012 Prompt: dz
      mask DialogControl ParameterTabVar0123 Prompt: Rx
      mask DialogControl ParameterTabVar01234 Prompt: Ry
      mask DialogControl ParameterTabVar012345 Prompt: Rz
  force : Outport
  des_pos : Outport  Port=2
  wires:
  Controller/1(force) -> force/1
  act_pos/1 -> Controller/1(act_pos)
  Inverse Kinematics Module/1(pos) -> Controller/3(des_pos), des_pos/1
  Inverse Kinematics Module/2(vel) -> Controller/4(des_vel)
  act_vel/1 -> Controller/2(act_vel)
  Reference Trajectory Generator1/1(d) -> Inverse Kinematics Module/1(d)
  Reference Trajectory Generator1/3(d') -> Inverse Kinematics Module/3(d')
  Reference Trajectory Generator1/4(R') -> Inverse Kinematics Module/4(R')
  Reference Trajectory Generator1/2(R) -> Inverse Kinematics Module/2(R)

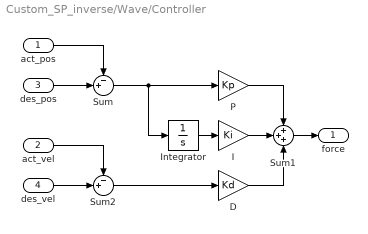
== system Custom_SP_inverse/Wave/Controller ==
  act_pos : Inport
  act_vel : Inport  Port=2
  des_pos : Inport  Port=3
  des_vel : Inport  Port=4
  D : Gain  Gain=Kd  SaturateOnIntegerOverflow=on  OutDataTypeStr=Inherit: Same as input  ParamDataTypeStr=Inherit: Same as input
  I : Gain  Gain=Ki  SaturateOnIntegerOverflow=on  OutDataTypeStr=Inherit: Same as input  ParamDataTypeStr=Inherit: Same as input
  Integrator : Integrator  ZeroCross=off
  P : Gain  Gain=Kp  SaturateOnIntegerOverflow=on  OutDataTypeStr=Inherit: Same as input  ParamDataTypeStr=Inherit: Same as input
  Sum : Sum  Inputs=-+|  InputSameDT=on  SaturateOnIntegerOverflow=on  OutDataTypeStr=Inherit: Same as first input
  Sum1 : Sum  Inputs=+++  InputSameDT=on  SaturateOnIntegerOverflow=on  OutDataTypeStr=Inherit: Same as first input
  Sum2 : Sum  Inputs=-+|  InputSameDT=on  SaturateOnIntegerOverflow=on  OutDataTypeStr=Inherit: Same as first input
  force : Outport  VectorParamsAs1DForOutWhenUnconnected=off
  wires:
  Sum2/1 -> D/1
  D/1 -> Sum1/3
  Integrator/1 -> I/1
  P/1 -> Sum1/1
  I/1 -> Sum1/2
  Sum/1 -> P/1, Integrator/1
  act_pos/1 -> Sum/1
  des_pos/1 -> Sum/2
  Sum1/1 -> force/1
  act_vel/1 -> Sum2/1
  des_vel/1 -> Sum2/2

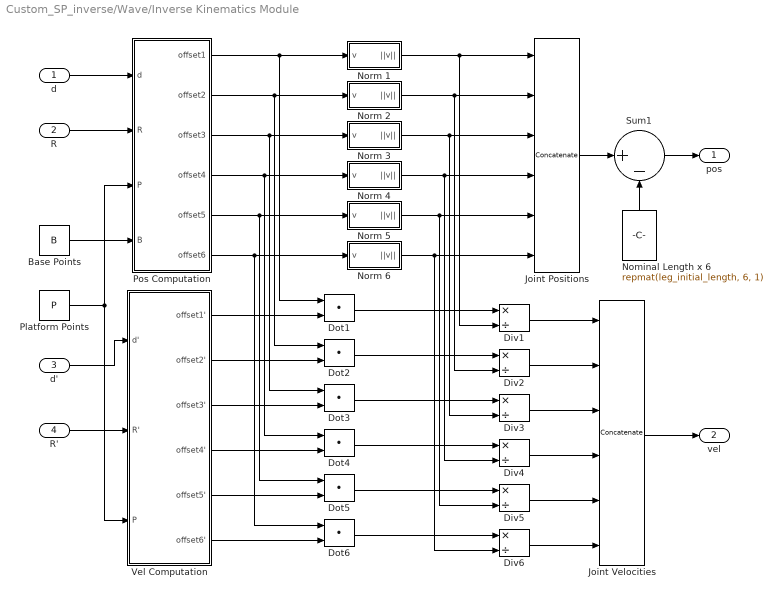
== system Custom_SP_inverse/Wave/Inverse Kinematics Module ==
  d : Inport
  R : Inport  Port=2
  d' : Inport  Port=3
  R' : Inport  Port=4
  Base Points : Constant  Value=B
  Div{1..6} (6 alike) : Product  Inputs=*/
  Dot{1..6} (6 alike) : DotProduct  OutDataTypeStr=Inherit: Inherit via internal rule
  Joint Positions : Concatenate  NumInputs=6  Mode=Multidimensional array
  Joint Velocities : Concatenate  NumInputs=6  Mode=Multidimensional array
  Nominal Length x 6 : Constant  Value=repmat(leg_initial_length, 6, 1)
  Norm 1 : Subsystem
  Norm 2 : Subsystem
  Norm 3 : Subsystem
  Norm 4 : Subsystem
  Norm 5 : Subsystem
  Norm 6 : Subsystem
  Platform Points : Constant  Value=P
  Pos Computation : Subsystem
  Sum1 : Sum  Inputs=|+-
  Vel Computation : Subsystem
  pos : Outport  VectorParamsAs1DForOutWhenUnconnected=off
  vel : Outport  Port=2  VectorParamsAs1DForOutWhenUnconnected=off
  wires:
  Joint Positions/1 -> Sum1/1
  Nominal Length x 6/1 -> Sum1/2
  Sum1/1 -> pos/1
  d/1 -> Pos Computation/1(d)
  R/1 -> Pos Computation/2(R)
  Base Points/1 -> Pos Computation/4(B)
  Platform Points/1 -> Vel Computation/3(P), Pos Computation/3(P)
  Pos Computation/4(offset4) -> Norm 4/1(v), Dot4/1
  Pos Computation/3(offset3) -> Norm 3/1(v), Dot3/1
  Pos Computation/2(offset2) -> Norm 2/1(v), Dot2/1
  Pos Computation/1(offset1) -> Norm 1/1(v), Dot1/1
  Pos Computation/5(offset5) -> Norm 5/1(v), Dot5/1
  Pos Computation/6(offset6) -> Norm 6/1(v), Dot6/1
  Norm 1/1(||v||) -> Joint Positions/1, Div1/2
  Norm 6/1(||v||) -> Joint Positions/6, Div6/2
  Norm 2/1(||v||) -> Joint Positions/2, Div2/2
  Norm 3/1(||v||) -> Joint Positions/3, Div3/2
  Norm 4/1(||v||) -> Joint Positions/4, Div4/2
  Norm 5/1(||v||) -> Joint Positions/5, Div5/2
  Vel Computation/3(offset3') -> Dot3/2
  Vel Computation/4(offset4') -> Dot4/2
  Vel Computation/2(offset2') -> Dot2/2
  Vel Computation/5(offset5') -> Dot5/2
  Vel Computation/6(offset6') -> Dot6/2
  d'/1 -> Vel Computation/1(d')
  Dot2/1 -> Div2/1
  Dot6/1 -> Div6/1
  Dot5/1 -> Div5/1
  Dot4/1 -> Div4/1
  Dot3/1 -> Div3/1
  Div1/1 -> Joint Velocities/1
  Div2/1 -> Joint Velocities/2
  Div6/1 -> Joint Velocities/6
  Div3/1 -> Joint Velocities/3
  Div4/1 -> Joint Velocities/4
  Div5/1 -> Joint Velocities/5
  Joint Velocities/1 -> vel/1
  R'/1 -> Vel Computation/2(R')
  Vel Computation/1(offset1') -> Dot1/2
  Dot1/1 -> Div1/1
